simulink library "sgtb_tlbx_1_0_2020b"  (R2020b)
settings: Solver=VariableStepAuto  StartTime=0.0  StopTime=10.0  RelTol=1e-3
libraries: $bdroot x30
settings Model: Creator=mne4  LastModifiedBy=mne4

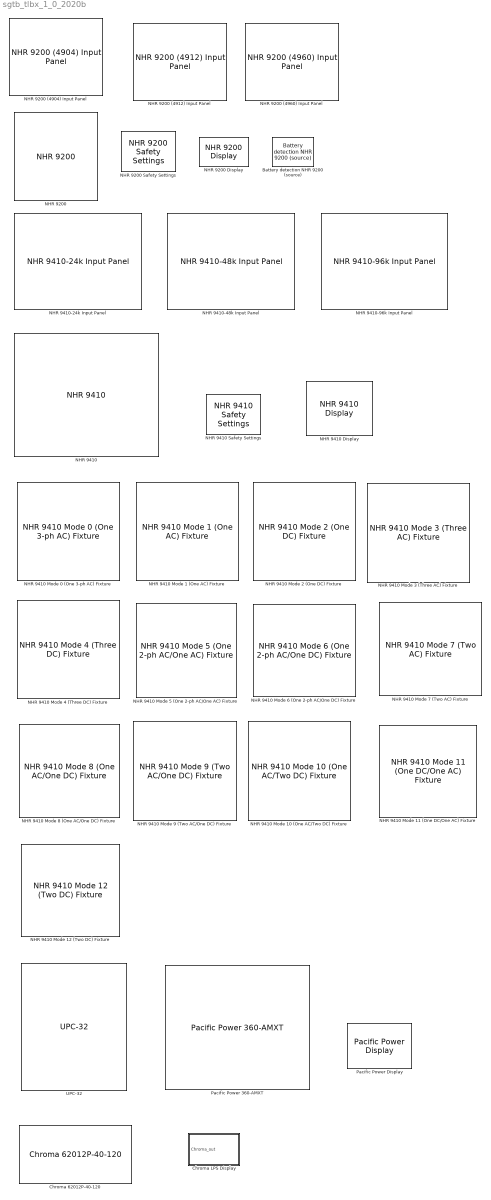
== system sgtb_tlbx_1_0_2020b ==
  Battery detection NHR 9200 (source) : $bdroot/Battery detection NHR 9200 (source)  Vdetect=0
  Chroma 62012P-40-120 : $bdroot/Chroma 62012P-40-120  set_out=1  v_out=30  i_out=20  Vmax=40  Vmin=0  Imax=120  Imin=0  Vslew=0.00001  Islew=0.00001  ttl=0  Vdcr=0  Vdcf=0  Vmax_prot=35  Imax_prot=125  Pmax_prot=1260
  Chroma LPS Display : Subsystem
      mask DialogControl ParameterGroupVar Prompt: NHR 9200 Display block
      mask DialogControl Control2 Prompt: Look under the mask for scopes and displays
  NHR 9200 : $bdroot/NHR 9200  p_switch=1  Vslew=200  Islew=100  Rslew=400  Pslew=300  Vbset=4
  NHR 9200 (4904) Input Panel : $bdroot/NHR 9200 (4904) Input Panel  op_state=2  Vmch=20  Imch=40.0  Pmch=8.0  Rsch=0.001  Vmdch=20  Imdch=40  Pmdch=12
  NHR 9200 (4912) Input Panel : $bdroot/NHR 9200 (4912) Input Panel  op_state=2  Vmch=100  Imch=40.0  Pmch=8.0  Rsch=0.001  Vmdch=20  Imdch=40  Pmdch=12
  NHR 9200 (4960) Input Panel : $bdroot/NHR 9200 (4960) Input Panel  op_state=2  Vmch=480.0  Imch=2  Pmch=8.0  Rsch=0.001  Vmdch=20  Imdch=40  Pmdch=12
  NHR 9200 Display : $bdroot/NHR 9200 Display  SystemSampleTime=-1  VariantActivationTime=update diagram  Latency=0  AutoFrameSizeCalculation=off
  NHR 9200 Safety Settings : $bdroot/NHR 9200 Safety Settings  Vmin=-50  Tvmin=2  Vmax=600  Tvmax=0.5  Imaxdch=80  Timaxdch=2  Pmaxdch=800  Tpmaxdch=2  Imaxch=10  Timaxch=0.5  Pmaxch=5000  Tpmaxch=2
  NHR 9410 : $bdroot/NHR 9410  p_switch=1  VslewAC=0.0  FslewAC=500.0  VslewDC=0.0  IslewDC=0.0  PslewDC=0.0
  NHR 9410 Display : $bdroot/NHR 9410 Display  SystemSampleTime=-1  VariantActivationTime=update diagram  Latency=0  AutoFrameSizeCalculation=off
  NHR 9410 Mode 0 (One 3-ph AC) Fixture : $bdroot/NHR 9410 Mode 0 (One 3-ph AC) Fixture  SystemSampleTime=-1  VariantActivationTime=update diagram  Latency=0  AutoFrameSizeCalculation=off
  NHR 9410 Mode 1 (One AC) Fixture : $bdroot/NHR 9410 Mode 1 (One AC) Fixture  SystemSampleTime=-1  VariantActivationTime=update diagram  Latency=0  AutoFrameSizeCalculation=off
  NHR 9410 Mode 10 (One AC/Two DC) Fixture : $bdroot/NHR 9410 Mode 10 (One AC//Two DC) Fixture  SystemSampleTime=-1  VariantActivationTime=update diagram  Latency=0  AutoFrameSizeCalculation=off
  NHR 9410 Mode 11 (One DC/One AC) Fixture : $bdroot/NHR 9410 Mode 11 (One DC//One AC) Fixture  SystemSampleTime=-1  VariantActivationTime=update diagram  Latency=0  AutoFrameSizeCalculation=off
  NHR 9410 Mode 12 (Two DC) Fixture : $bdroot/NHR 9410 Mode 12 (Two DC) Fixture  SystemSampleTime=-1  VariantActivationTime=update diagram  Latency=0  AutoFrameSizeCalculation=off
  NHR 9410 Mode 2 (One DC) Fixture : $bdroot/NHR 9410 Mode 2 (One DC) Fixture  SystemSampleTime=-1  VariantActivationTime=update diagram  Latency=0  AutoFrameSizeCalculation=off
  NHR 9410 Mode 3 (Three AC) Fixture : $bdroot/NHR 9410 Mode 3 (Three AC) Fixture  SystemSampleTime=-1  VariantActivationTime=update diagram  Latency=0  AutoFrameSizeCalculation=off
  NHR 9410 Mode 4 (Three DC) Fixture : $bdroot/NHR 9410 Mode 4 (Three DC) Fixture  SystemSampleTime=-1  VariantActivationTime=update diagram  Latency=0  AutoFrameSizeCalculation=off
  NHR 9410 Mode 5 (One 2-ph AC/One AC) Fixture : $bdroot/NHR 9410 Mode 5 (One 2-ph AC//One AC) Fixture  SystemSampleTime=-1  VariantActivationTime=update diagram  Latency=0  AutoFrameSizeCalculation=off
  NHR 9410 Mode 6 (One 2-ph AC/One DC) Fixture : $bdroot/NHR 9410 Mode 6 (One 2-ph AC//One DC) Fixture  SystemSampleTime=-1  VariantActivationTime=update diagram  Latency=0  AutoFrameSizeCalculation=off
  NHR 9410 Mode 7 (Two AC) Fixture : $bdroot/NHR 9410 Mode 7 (Two AC) Fixture  SystemSampleTime=-1  VariantActivationTime=update diagram  Latency=0  AutoFrameSizeCalculation=off
  NHR 9410 Mode 8 (One AC/One DC) Fixture : $bdroot/NHR 9410 Mode 8 (One AC//One DC) Fixture  SystemSampleTime=-1  VariantActivationTime=update diagram  Latency=0  AutoFrameSizeCalculation=off
  NHR 9410 Mode 9 (Two AC/One DC) Fixture : $bdroot/NHR 9410 Mode 9 (Two AC//One DC) Fixture  SystemSampleTime=-1  VariantActivationTime=update diagram  Latency=0  AutoFrameSizeCalculation=off
  NHR 9410 Safety Settings : $bdroot/NHR 9410 Safety Settings  Vmin1=-50  Tvmin1=2  Svmin1=-1  Vmax1=100  Tvmax1=0.2  Svmax1=-1  Vpeak1=100  Vpeaken1=0  Imaxsrc1=80  Timaxsrc1=2  Simaxsrc1=-1  Imaxsnk1=50  Timaxsnk1=2  Simaxsnk1=-1  Ipeak1=80  Ipeaken1=0  Pmaxsrc1=2000  Tpmaxsrc1=2  Spmaxsrc1=-1  Pmaxsnk1=50  Tpmaxsnk1=2  Spmaxsnk1=-1  Vmin2=-50  Tvmin2=2  Svmin2=-1  Vmax2=90  Tvmax2=0.5  Svmax2=-1  Vpeak2=80  Vpeaken2=0  Imaxsrc2=50  Timaxsrc2=2  Simaxsrc2=-1  Imaxsnk2=8  Timaxsnk2=5  Simaxsnk2=1  Ipeak2=80  Ipeaken2=0  Pmaxsrc2=50  Tpmaxsrc2=2  Spmaxsrc2=-1  Pmaxsnk2=50  Tpmaxsnk2=2  Spmaxsnk2=-1  Vmin3=-50  Tvmin3=2  Svmin3=-1  Vmax3=500  Tvmax3=0.5  Svmax3=-1  Vpeak3=80  Vpeaken3=0  Imaxsrc3=50  Timaxsrc3=2  Simaxsrc3=-1  Imaxsnk3=8  Timaxsnk3=0.2  Simaxsnk3=-1  Ipeak3=80  Ipeaken3=0  Pmaxsrc3=50  Tpmaxsrc3=2  Spmaxsrc3=-1  Pmaxsnk3=3000  Tpmaxsnk3=0.2  Spmaxsnk3=1
  NHR 9410-24k Input Panel : $bdroot/NHR 9410-24k Input Panel  sel=6  md0Pm1=20  md0Vrms1=277  md0Irms1=100  md0f1=60  md1Pm=20  md1Vrms=277  md1Irms=100  md1f=60  md1ph=0  md2Pm=20  md2Vm=400  md2Im=100  md3Pm1=5  md3Vrms1=277  md3Irms1=50  md3f1=60  md3ph1=0.0  md3Pm2=5  md3Vrms2=277  md3Irms2=50  md3f2=60  md3ph2=0  md3Pm3=20  md3Vrms3=277  md3Irms3=50  md3f3=60  md3ph3=0  md4Pm1=5  md4Vm1=400  md4Im1=50  md4Pm2=5  md4Vm2=400.0  md4Im2=50  md4Pm3=5  md4Vm3=400.0  md4Im3=50  md5Pm1=10  md5Vrms1=500  md5Irms1=50  md5f1=60  md5Pm2=5  md5Vrms2=350.0  md5Irms2=50  md5f2=60  md5ph2=0  md6Pm1=10  md6Vrms1=215.0  md6Irms1=50  md6f1=60  md6Pm2=5  md6Vm2=400.0  md6Im2=50  md7Pm1=10  md7Vrms1=277  md7Irms1=100  md7f1=60  md7ph1=0  md7Pm2=5  md7Vrms2=277  md7Irms2=50  md7f2=60  md7ph2=0  md8Pm1=10  md8Vrms1=277  md8Irms1=100  md8f1=60  md8ph1=0  md8Pm2=5  md8Vm2=400  md8Im2=50  md9Pm1=5  md9Vrms1=224.0  md9Irms1=50  md9f1=60  md9ph1=0  md9Pm2=5  md9Vrms2=277  md9Irms2=50  md9f2=60  md9ph2=0  md9Pm3=5  md9Vm3=400.0  md9Im3=50  md10Pm1=5  md10Vrms1=277  md10Irms1=50  md10f1=60  md10ph1=0  md10Pm2=5  md10Vm2=50  md10Im2=50  md10Pm3=5  md10Vm3=392.0  md10Im3=50  md11Pm1=10  md11Vm1=400.0  md11Im1=100  md11Pm2=5  md11Vrms2=277  md11Irms2=50  md11f2=60  md11ph2=0  md12Pm1=10  md12Vm1=400.0  md12Im1=100  md12Pm2=5  md12Vm2=400.0  md12Im2=50
  NHR 9410-48k Input Panel : $bdroot/NHR 9410-48k Input Panel  sel=6  md0Pm1=40  md0Vrms1=277  md0Irms1=100  md0f1=60  md1Pm=40  md1Vrms=277  md1Irms=300  md1f=60  md1ph=0  md2Pm=40  md2Vm=400  md2Im=300  md3Pm1=10  md3Vrms1=277  md3Irms1=100  md3f1=60  md3ph1=0.0  md3Pm2=10  md3Vrms2=277  md3Irms2=100  md3f2=60  md3ph2=0  md3Pm3=10  md3Vrms3=277  md3Irms3=100  md3f3=60  md3ph3=0  md4Pm1=10  md4Vm1=400  md4Im1=100  md4Pm2=10  md4Vm2=400.0  md4Im2=100  md4Pm3=10  md4Vm3=400.0  md4Im3=100  md5Pm1=30  md5Vrms1=500  md5Irms1=100  md5f1=60  md5Pm2=10  md5Vrms2=350.0  md5Irms2=100  md5f2=60  md5ph2=0  md6Pm1=30  md6Vrms1=215.0  md6Irms1=100  md6f1=60  md6Pm2=10  md6Vm2=400.0  md6Im2=100  md7Pm1=30  md7Vrms1=277  md7Irms1=200  md7f1=60  md7ph1=0  md7Pm2=10  md7Vrms2=277  md7Irms2=100  md7f2=60  md7ph2=0  md8Pm1=30  md8Vrms1=277  md8Irms1=200  md8f1=60  md8ph1=0  md8Pm2=10  md8Vm2=400  md8Im2=100  md9Pm1=10  md9Vrms1=224.0  md9Irms1=100  md9f1=60  md9ph1=0  md9Pm2=10  md9Vrms2=277  md9Irms2=100  md9f2=60  md9ph2=0  md9Pm3=10  md9Vm3=400.0  md9Im3=100  md10Pm1=10  md10Vrms1=277  md10Irms1=100  md10f1=60  md10ph1=0  md10Pm2=10  md10Vm2=50  md10Im2=100  md10Pm3=10  md10Vm3=392.0  md10Im3=100  md11Pm1=30  md11Vm1=400.0  md11Im1=200  md11Pm2=10  md11Vrms2=277  md11Irms2=100  md11f2=60  md11ph2=0  md12Pm1=30  md12Vm1=400.0  md12Im1=200  md12Pm2=10  md12Vm2=400.0  md12Im2=100
  NHR 9410-96k Input Panel : $bdroot/NHR 9410-96k Input Panel  sel=3  md0Pm1=80  md0Vrms1=277  md0Irms1=199.200  md0f1=60  md1Pm=96.0  md1Vrms=277  md1Irms=720.0  md1f=60  md1ph=0  md2Pm=96  md2Vm=400  md2Im=720  md3Pm1=20  md3Vrms1=277  md3Irms1=200  md3f1=60  md3ph1=0.0  md3Pm2=20  md3Vrms2=277  md3Irms2=200  md3f2=60  md3ph2=0  md3Pm3=20  md3Vrms3=277  md3Irms3=200  md3f3=60  md3ph3=0  md4Pm1=32  md4Vm1=400  md4Im1=232.800  md4Pm2=32.0  md4Vm2=400.0  md4Im2=240.0  md4Pm3=32.0  md4Vm3=400.0  md4Im3=240.0  md5Pm1=64.0  md5Vrms1=500  md5Irms1=240.0  md5f1=60  md5Pm2=32.0  md5Vrms2=350.0  md5Irms2=240.0  md5f2=60  md5ph2=0  md6Pm1=64  md6Vrms1=215.0  md6Irms1=240.0  md6f1=60  md6Pm2=32.0  md6Vm2=400.0  md6Im2=240.0  md7Pm1=64.0  md7Vrms1=277  md7Irms1=480.0  md7f1=60  md7ph1=0  md7Pm2=32.0  md7Vrms2=277  md7Irms2=240.0  md7f2=60  md7ph2=0  md8Pm1=32  md8Vrms1=277  md8Irms1=200  md8f1=60  md8ph1=0  md8Pm2=32  md8Vm2=400  md8Im2=200  md9Pm1=26.560  md9Vrms1=224.0  md9Irms1=240.0  md9f1=60  md9ph1=0  md9Pm2=32.0  md9Vrms2=277  md9Irms2=240.0  md9f2=60  md9ph2=0  md9Pm3=32.0  md9Vm3=400.0  md9Im3=240.0  md10Pm1=32.0  md10Vrms1=277  md10Irms1=237.600  md10f1=60  md10ph1=0  md10Pm2=2.240  md10Vm2=50  md10Im2=14.400  md10Pm3=31.680  md10Vm3=392.0  md10Im3=240.0  md11Pm1=64.0  md11Vm1=400.0  md11Im1=480.0  md11Pm2=32.0  md11Vrms2=277  md11Irms2=240.0  md11f2=60  md11ph2=0  md12Pm1=64  md12Vm1=400.0  md12Im1=480.0  md12Pm2=32.0  md12Vm2=400.0  md12Im2=240.0
  Pacific Power 360-AMXT : $bdroot/Pacific Power 360-AMXT  p_switch=1  VslewAC=5.000e+05  FslewAC=500.0  VslewDC=20000.0  IslewDC=1.000e+05  PslewDC=1.000e+06
  Pacific Power Display : $bdroot/Pacific Power Display  SystemSampleTime=-1  VariantActivationTime=update diagram  Latency=0  AutoFrameSizeCalculation=off
  UPC-32 : $bdroot/UPC-32  f=60  sel=1  form_sel=2  Vm11=100  Im11=10  Vm12=100  Im12=10  Vm13a=100  Vm13b=100  Vm13c=100  Ph13b=120  Ph13c=240  Im13=10  Vm21=100  Im21=0  Vm22=100  Im22=0  Vm23a=100  Vm23b=100  Vm23c=100  Ph23b=120  Ph23c=240  Im23=10  Zout=10  Iprt=0  Iprtlim=0  Tiprt=0

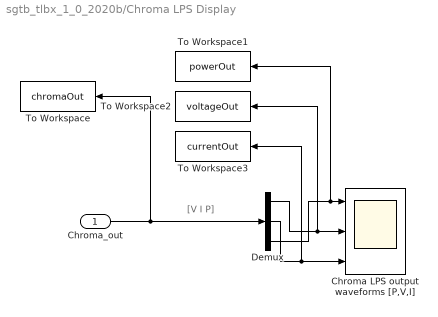
== system sgtb_tlbx_1_0_2020b/Chroma LPS Display ==
  note: [V I P]
  Chroma_out : Inport
  Chroma LPS output waveforms [P,V,I] : Scope  NumInputPorts=3
  Demux : Demux  Outputs=3
  To Workspace : ToWorkspace  VariableName=chromaOut  SaveFormat=Timeseries  SampleTime=-1
  To Workspace1 : ToWorkspace  VariableName=powerOut  SaveFormat=Timeseries  SampleTime=-1
  To Workspace2 : ToWorkspace  VariableName=voltageOut  SaveFormat=Timeseries  SampleTime=-1
  To Workspace3 : ToWorkspace  VariableName=currentOut  SaveFormat=Timeseries  SampleTime=-1
  wires:
  Chroma_out/1 -> To Workspace/1, Demux/1
  Demux/3 -> To Workspace1/1, Chroma LPS output waveforms [P,V,I]/1
  Demux/1 -> To Workspace2/1, Chroma LPS output waveforms [P,V,I]/2
  Demux/2 -> To Workspace3/1, Chroma LPS output waveforms [P,V,I]/3
